simulink model "Pacemaker"  (R2022a)
settings: Solver=VariableStepAuto  StartTime=0.0  StopTime=10.0  RelTol=1e-3
libraries: simulink x1
settings Model: Creator=bkfre  LastModifiedBy=Aldraech
settings DebuggingCC: UnconnectedInputMsg=warning  UnconnectedOutputMsg=warning  UnconnectedLineMsg=warning
settings RTWCC: DLArmComputeVersion=19.05

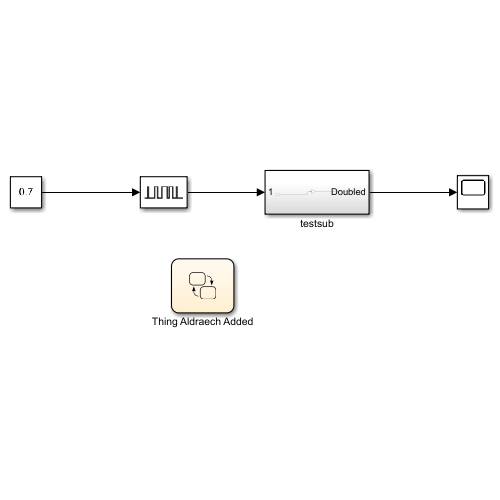
[thumbnail: Simulink's stored preview of the top-level diagram]
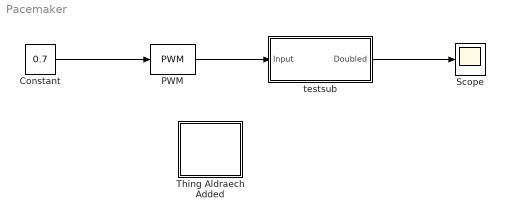
== system Pacemaker ==
  Constant : Constant  Value=0.7
  PWM : simulink/Discontinuities/PWM  DisableCoverage=on  Period=0.5  DisallowZeroDutyCycle=off  RunAtFixedTimeIntervals=off  SampleTime=0.1
  Scope : Scope
  Thing Aldraech Added : Stateflow chart  TreatAsAtomicUnit=on
  testsub : Subsystem
  wires:
  Constant/1 -> PWM/1
  PWM/1 -> testsub/1(Input)
  testsub/1(Doubled) -> Scope/1

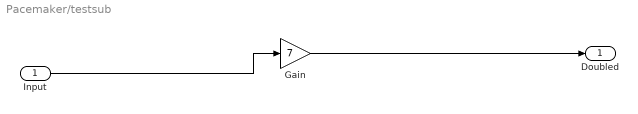
== system Pacemaker/testsub ==
  Input : Inport
  Gain : Gain  Gain=7
  Doubled : Outport
  wires:
  Input/1 -> Gain/1
  Gain/1 -> Doubled/1

== stateflow chart Pacemaker/Thing Aldraech Added ==
